simulink model "modelo_f_nico_local"  (R2024b)
settings: Solver=ode15s  StartTime=0.0  StopTime=600  FixedStep=0.001  RelTol=1e-3
InitFcn:
  | clc
  | clear
  | close all
  | parametros
  | gain_CL
  | calculo_observador_carro
  | calculo_observador_izaje
values from neighbouring files (symbols this model uses):
  b_cx = 1e6    (= 1000000)    [parametros.m]
  b_cy = 1e7    (= 10000000)    [parametros.m]
  b_ha = -(J_hEq + (r_hd/(2*i_h))*m_l) * w_des_h*(1 + n_h + n_h^2) + b_hEq    [gain_CL.m]
  b_hb = 1e8    (= 100000000)    [parametros.m]
  b_hd = 8    [parametros.m]
  b_hm = 18    [parametros.m]
  b_t = 90    [parametros.m]
  b_ta = M_tEq*w_des_t*(1+n_t+n_t^2)-b_tEq    [gain_CL.m]
  b_tb = 5e6    (= 5000000)    [parametros.m]
  b_td = 1.8    [parametros.m]
  b_tm = 6    [parametros.m]
  b_tw = 3e3    (= 3000)    [parametros.m]
  b_wu = 150    [parametros.m]
  g = 9.80665    [parametros.m]
  H_c = 2.59    [parametros.m]
  i_h = 22    [parametros.m]
  i_t = 30    [parametros.m]
  J_hd_hEb = 3800    [parametros.m]
  J_hm_hb = 30    [parametros.m]
  J_td = 1200    [parametros.m]
  J_tm_tb = 7    [parametros.m]
  K_cy = 1.8e9    (= 1800000000)    [parametros.m]
  k_hsa = -(J_hEq + (r_hd/(2*i_h))*m_l) * w_des_h^2*(n_h + n_h^2 + n_h^3)    [gain_CL.m]
  k_hsia = -(J_hEq + (r_hd/(2*i_h))*m_l) * n_h^3 * w_des_h^3    [gain_CL.m]
  k_tsa = M_tEq*w_des_t^2*n_t*(1+n_t+n_t^2)    [gain_CL.m]
  k_tsia = M_tEq*w_des_t^3*n_t^3    [gain_CL.m]
  K_tw = 4.8e5    (= 480000)    [parametros.m]
  k_wu = 2.36e8    (= 236000000)    [parametros.m]
  l_h_max = Y_t0-y_h_min    (= 65)    [parametros.m]
  l_h_maxE = l_h_max+0.5    (= 65.5)    [parametros.m]
  l_h_min = Y_t0-y_h_max    (= 5)    [parametros.m]
  l_h_minE = l_h_min-0.5    (= 4.5)    [parametros.m]
  Lt = place(At', Ct', polos_deseados)'    [calculo_observador_carro.m]
  M_cmax = 50000    [parametros.m]
  M_cmin = 2000    [parametros.m]
  M_s = 15000    [parametros.m]
  M_t = 30000    [parametros.m]
  r_hd = 0.75    [parametros.m]
  r_td = 0.50    (= 0.5)    [parametros.m]
  T_hbMax = 5e4    (= 50000)    [parametros.m]
  T_hEbMax = 1.1e6    (= 1100000)    [parametros.m]
  T_hmMax = 2e4    (= 20000)    [parametros.m]
  T_s = 0.001    [parametros.m]
  T_tbMax = 5e3    (= 5000)    [parametros.m]
  T_tmMax = 4e3    (= 4000)    [parametros.m]
  tau_tm = 1e-3    (= 0.001)    [parametros.m]
  tau_wl = 1 / (2 * pi * 2)    (= 0.0795774715459)    [parametros.m]
  theta_hm0 = -l_h0*i_h*2/r_hd    (= -2229.33333333)    [parametros.m]
  theta_tm0 = (x_t0)*i_t/r_td    (= -900)    [parametros.m]
  v_h_max_noload = 3    [parametros.m]
  v_lx0 = 0    [parametros.m]
  v_ly0 = 0    [parametros.m]
  v_t0 = 0    [parametros.m]
  v_t_max = 4    [parametros.m]
  W_c = ctrb(A, B_c(:,1))    [CyO_carro.m]    (also in CyO_izaje.m; parametros.m = 2.44)
  w_hm0 = 0    [parametros.m]
  w_hm_min_BRK = 999999999    [parametros.m]
  w_hm_rated = v_h_max_load*2*i_h/r_hd    (= 88)    [parametros.m]
  w_tm0 = (v_t0)*i_t/r_td    (= 0)    [parametros.m]
  w_tm_min_BRK = 999999999    [parametros.m]
  x_l0 = x_t0    (= -15)    [parametros.m]
  x_lidar_offset = 3.0    (= 3)    [parametros.m]
  x_t0 = -15    [parametros.m]
  x_t_max = 50    [parametros.m]
  x_t_maxE = x_t_max+0.5    (= 50.5)    [parametros.m]
  x_t_min = -30    [parametros.m]
  x_t_minE = x_t_min-0.5    (= -30.5)    [parametros.m]
  y_h_min = -20    [parametros.m]
  y_l0 = 7    [parametros.m]
  Y_sb = 5.0    (= 5)    [parametros.m]
  Y_t0 = 45    [parametros.m]
undefined symbols (not defined in the file or in its folder): carro_FC_safety_margin, izaje_FC_safety_margin, Lh
libraries: dspsigops x1, simulink x1
(part 1 of 2)
settings Model: Creator=nsorr  LastModifiedBy=nsorr
settings SolverCC: DecoupledContinuousIntegration=on

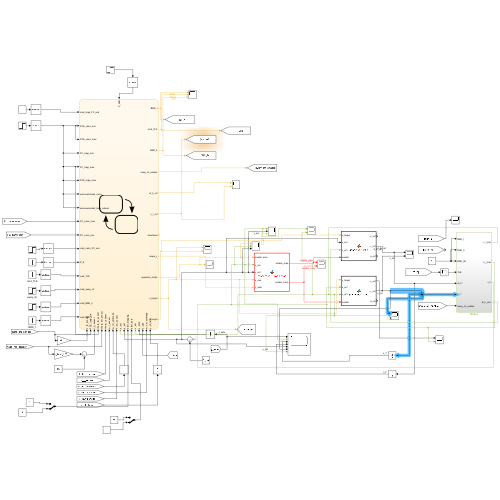
[thumbnail: Simulink's stored preview of the top-level diagram]
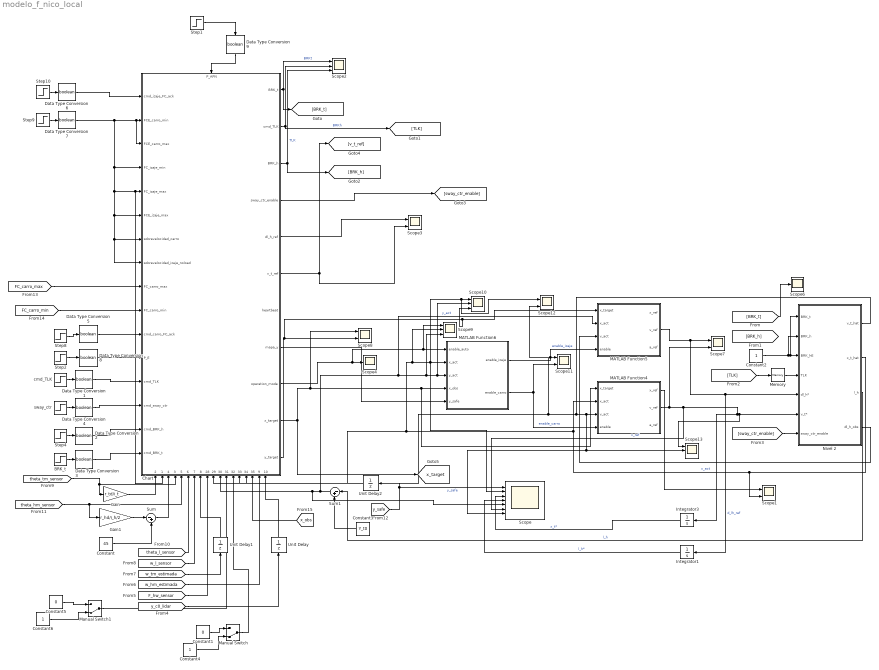
== system modelo_f_nico_local ==
  BRK_t : Step  Time=0  After=0  SampleTime=0
  Chart : Stateflow chart  TreatAsAtomicUnit=on
      settings: PortSchema="{\"entries\":[{\"content\":{\"sides\":[{\"content\":{\"connectorIds\":[\"In15\",\"In16\",\"In17\",\"In18\",\"In19\",\"In20\",\"In21\",\"In22\",\"In23\",\"In24\",\"In13\",\"In12\",\"In25\",\"In14\",\"In26\",\"In27\"]},\"type\":\"ConnectorPlacement.EquallySpacedRectSide\",\"uuid\":\"7880b9cd-08fb-4733-bb6b-48e405180dc5\"},{\"content\":{\"connectorIds\":[\"Out1\",\"Out3\",\"Out4\",\"Out5\",\"Out6\",\"Out2\",\"Out7\",\"Out8\",\"Out9\",\"Out10\",\"Out11\"],\"side\":\"RIGHT\"},\"type\":\"ConnectorPlacement.EquallySpacedRectSide\",\"uuid\":\"1a0088c7-0ec1-46fb-bd67-3069194311ce\"},{\"content\":{\"connectorIds\":[\"In11\"],\"side\":\"TOP\"},\"type\":\"ConnectorPlacement.EquallySpacedRectSide\",\"uuid\":\"63c24ea1-9c7d-47d6-85d5-bbef0a7be167\"},{\"content\":{\"connectorIds\":[\"In2\",\"In1\",\"In4\",\"In3\",\"In5\",\"In6\",\"In7\",\"In8\",\"In28\",\"In29\",\"In30\",\"In31\",\"In32\",\"In33\",\"In34\",\"In35\",\"In9\",\"In10\"],\"side\":\"BOTTOM\"},\"type\":\"ConnectorPlacement.EquallySpacedRectSide\",\"uuid\":\"56586e70-7155-4caa-800e-4bb67e399bfa\"}]},\"type\":\"ConnectorPlacement.EquallySpacedConnector\",\"uuid\":\"e7da0abc-eae0-41d9-ad4b-a3df1daa3702\"}],\"packageUris\":[\"http://schema.mathworks.com/mf0/Connector/R2020b\"],\"version\":\"1.0\"}"
  Constant : Constant  Value=45
  Constant1 : Constant  Value=0  OutDataTypeStr=boolean
  Constant2 : Constant
  Constant3 : Constant  Value=Y_t0
  Constant4 : Constant  OutDataTypeStr=boolean
  Constant5 : Constant  Value=0  OutDataTypeStr=boolean
  Constant6 : Constant  OutDataTypeStr=boolean
  Data Type Conversion{1..9} (9 alike) : DataTypeConversion  OutDataTypeStr=boolean  SaturateOnIntegerOverflow=off  RndMeth=Floor
  Gain : Gain  Gain=r_td/i_t
  Gain1 : Gain  Gain=r_hd/i_h/2
  Integrator1 : Integrator  InitialCondition=x_t0
  Integrator3 : Integrator  InitialCondition=x_t0
  MATLAB Function4 : MATLAB Function  TreatAsAtomicUnit=on  SystemSampleTime=T_s
  MATLAB Function5 : MATLAB Function  TreatAsAtomicUnit=on  SystemSampleTime=T_s
  MATLAB Function6 : MATLAB Function  TreatAsAtomicUnit=on  SystemSampleTime=T_s
  Manual Switch : ManualSwitch  CurrentSetting=0
  Manual Switch1 : ManualSwitch  CurrentSetting=0
  Memory : Memory
  Nivel 2 : Subsystem
  Scope : Scope  NumInputPorts=7
  Scope{1,3,7..8,11..12} (6 alike) : Scope  NumInputPorts=2
  Scope{2,9..10,13} (4 alike) : Scope  NumInputPorts=3
  Scope4 : Scope
  Scope6 : Scope
  Step1 : Step  SampleTime=0
  Step{4,8..10} (4 alike) : Step  Time=0  After=0  SampleTime=0
  Step2 : Step  Time=0  SampleTime=0
  Sum : Sum  Inputs=|-+
  Sum1 : Sum  Inputs=|-+
  Unit Delay : UnitDelay  SampleTime=T_s  HasFrameUpgradeWarning=on
  Unit Delay1 : UnitDelay  SampleTime=T_s  HasFrameUpgradeWarning=on
  Unit Delay2 : UnitDelay  SampleTime=T_s  HasFrameUpgradeWarning=on
  cmd_TLK : Step  Time=0  After=0  SampleTime=0
  sway_ctr : Step  Time=0  After=0  SampleTime=0
  tag scope: x_target=global
  wires:
  MATLAB Function5/2(v_ref) -> Scope7/1, Nivel 2/5(dl_h*), Integrator1/1  "d_lh_ref"
  Chart/9(operation_mode) -> Scope9/1, MATLAB Function6/1(enable_auto), Scope4/1
  Chart/1(BRK_t) -> [BRK_t], Scope2/1  "BRKt"
  [F_hw_sensor] -> Chart/28(F_hw_sensor)
  [theta_tm_sensor] -> Gain/1, Chart/3(theta_tm_sensor)
  [FC_carro_max] -> Chart/23(FC_carro_max)
  cmd_TLK/1 -> Data Type Conversion1/1
  Gain1/1 -> Sum/1
  Chart/6(dl_h_ref) -> Scope3/1
  Data Type Conversion7/1 -> Chart/17(FCE_carro_max), Chart/16(FCE_carro_min), Chart/18(FC_izaje_min), Chart/19(FC_izaje_max), Chart/1(FCE_izaje_min), Chart/22(sobrevelocidad_izaje_noload), Chart/21(sobrevelocidad_carro), Chart/20(FCE_izaje_max)
  Step2/1 -> Data Type Conversion8/1
  [theta_l_sensor] -> Chart/6(theta_l_sensor)
  Constant3/1 -> Sum1/2
  Chart/4(BRK_h) -> Scope2/3, [BRK_h]  "TLK"
  Data Type Conversion9/1 -> Chart/11(P_APN)
  Constant/1 -> Sum/2
  Gain/1 -> Chart/2(x_td_sensor)
  MATLAB Function6/2(enable_carro) -> Scope11/2, MATLAB Function4/4(enable)  "enable_carro"
  Data Type Conversion2/1 -> Chart/26(cmd_BRK_h)
  Step4/1 -> Data Type Conversion2/1
  [w_tm_estimada] -> Unit Delay1/1
  Manual Switch1/1 -> Chart/31(start_mapping)
  sway_ctr/1 -> Data Type Conversion4/1
  [w_hm_estimada] -> Chart/9(w_hm_estimada)
  Unit Delay1/1 -> Chart/8(w_tm_estimada)
  Sum1/1 -> MATLAB Function5/2(x_act), Scope10/2, MATLAB Function6/3(y_act), Scope9/3, Scope/5, Chart/30(y_act)  "y_act"
  Nivel 2/1(v_t_hat) -> Scope12/2, Chart/33(v_act), Scope13/2, Scope/7, MATLAB Function4/3(v_act)
  Chart/5(sway_ctr_enable) -> [sway_ctr_enable]
  [TLK] -> Memory/1
  [w_l_sensor] -> Chart/7(w_l_sensor)
  [BRK_t] -> Scope6/1
  Chart/2(v_t_ref) -> [v_t_ref], Scope3/2
  Data Type Conversion8/1 -> Chart/12(P_E)
  [theta_hm_sensor] -> Chart/5(theta_hm_sensor), Gain1/1
  Nivel 2/4(dl_h_obs) -> MATLAB Function5/3(v_act)
  Sum/1 -> Chart/4(l_h_sensor)
  [sway_ctr_enable] -> Nivel 2/7(sway_ctr_enable)
  Data Type Conversion1/1 -> Chart/25("cmd_TLK ")
  Nivel 2/3(l_h) -> Sum1/1  "l_h"
  Unit Delay/1 -> Chart/10(y_c0_lidar)
  Data Type Conversion5/1 -> Chart/13(cmd_carro_FC_ack)
  Nivel 2/2(x_t_hat) -> Scope1/2, MATLAB Function4/2(x_act), Chart/29(x_act), Scope12/1, Scope10/1, Scope/2, MATLAB Function6/2(x_act), Scope9/2  "x_act"
  Data Type Conversion6/1 -> Chart/15(cmd_izaje_FC_ack)
  Constant2/1 -> Nivel 2/1(BRK_t), Nivel 2/3(BRK_hE), Nivel 2/2(BRK_h)
  Step10/1 -> Data Type Conversion6/1
  MATLAB Function6/1(enable_izaje) -> MATLAB Function5/4(enable), Scope11/1  "enable_izaje"
  [y_c0_lidar] -> Unit Delay/1
  Chart/8(mapa_y) -> MATLAB Function6/5(y_safe)
  BRK_t/1 -> Data Type Conversion3/1
  Step8/1 -> Data Type Conversion5/1
  Chart/11(y_target) -> Scope8/2, Scope10/3, MATLAB Function5/1(x_target)
  Data Type Conversion4/1 -> Chart/14(cmd_sway_ctr)
  Step1/1 -> Data Type Conversion9/1
  Chart/10(x_target) -> Scope8/1, MATLAB Function4/1(x_target), MATLAB Function6/4(x_obs), [x_target]
  Data Type Conversion3/1 -> Chart/27(cmd_BRK_t)
  Step9/1 -> Data Type Conversion7/1
  Chart/3(cmd_TLK) -> [TLK], Scope2/2  "BRKh"
  MATLAB Function4/2(v_ref) -> Scope/6, Nivel 2/6(v_t*), Scope13/1, Integrator3/1, Scope7/2  "v_ref"
  [FC_carro_min] -> Chart/24(FC_carro_min)
  [y_safe] -> Unit Delay2/1, Scope/1  "y_safe"
  Unit Delay2/1 -> Chart/34(y_safe)
  Constant1/1 -> Manual Switch/1
  Constant4/1 -> Manual Switch/2
  Manual Switch/1 -> Chart/32(start_auto)
  Constant6/1 -> Manual Switch1/2
  Constant5/1 -> Manual Switch1/1
  Integrator3/1 -> Scope/3  "x_t*"
  Integrator1/1 -> Scope/4  "l_h*"
  [x_obs] -> Chart/35(x_obs)
  Memory/1 -> Nivel 2/4(TLK)
  MATLAB Function4/1(x_ref) -> Scope1/1

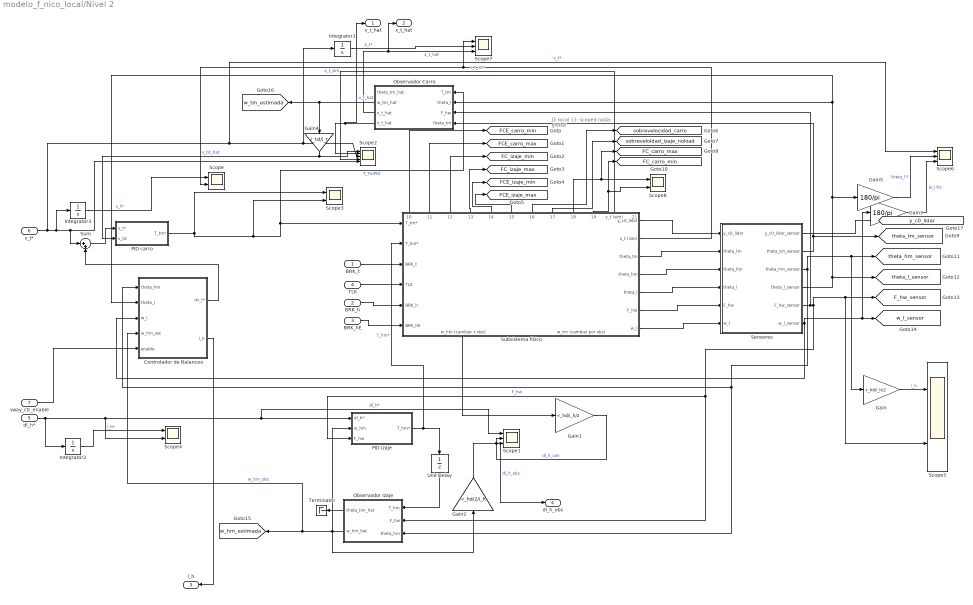
== system modelo_f_nico_local/Nivel 2 ==
  note: []: local
      | {}: scoped
      | nada: global
  BRK_t : Inport
  BRK_h : Inport  Port=2
  BRK_hE : Inport  Port=3
  TLK : Inport  Port=4
  dl_h* : Inport  Port=5
  v_t* : Inport  Port=6
  sway_ctr_enable : Inport  Port=7
  Controlador de Balanceo : Subsystem
  Gain : Gain  Gain=-r_hd/i_h/2
  Gain1 : Gain  Gain=-r_hd/i_h/2
  Gain2 : Gain  Gain=-r_hd/2/i_h
  Gain3 : Gain  Gain=180/pi
  Gain4 : Gain  Gain=r_td/i_t
  Gain5 : Gain  Gain=180/pi
  Integrator1 : Integrator  InitialCondition=x_t0
  Integrator2 : Integrator
  Integrator3 : Integrator  InitialCondition=x_t0
  Observador Carro : Subsystem
  Observador Izaje : Subsystem
  PID carro : Subsystem
  PID izaje : Subsystem
  Scope{,3..5,8} (5 alike) : Scope  NumInputPorts=2
  Scope1 : Scope  NumInputPorts=3
  Scope2 : Scope  NumInputPorts=5
  Scope6 : Scope  NumInputPorts=3
  Scope7 : Scope  NumInputPorts=3
  Sensores : Subsystem
  Subsistema físico : Subsystem
      settings: PortSchema="{\"entries\":[{\"content\":{\"sides\":[{\"content\":{\"connectorIds\":[\"In1\",\"In2\",\"In3\",\"In4\",\"In5\",\"In6\"]},\"type\":\"ConnectorPlacement.EquallySpacedRectSide\",\"uuid\":\"aa1cb789-2051-45a4-8cb8-6dd2078290cc\"},{\"content\":{\"connectorIds\":[\"Out1\",\"Out2\",\"Out3\",\"Out4\",\"Out5\",\"Out6\",\"Out7\"],\"side\":\"RIGHT\"},\"type\":\"ConnectorPlacement.EquallySpacedRectSide\",\"uuid\":\"7fe62279-dd3b-46db-ba9e-e4633dcea5c6\"},{\"content\":{\"connectorIds\":[\"Out10\",\"Out11\",\"Out12\",\"Out13\",\"Out14\",\"Out15\",\"Out16\",\"Out17\",\"Out18\",\"Out19\",\"Out20\",\"Out21\"],\"side\":\"TOP\"},\"type\":\"ConnectorPlacement.EquallySpacedRectSide\",\"uuid\":\"a5663ea7-10d8-47d7-b8ed-8fbfb239b85a\"},{\"content\":{\"connectorIds\":[\"Out8\",\"Out9\"],\"side\":\"BOTTOM\"},\"type\":\"ConnectorPlacement.EquallySpacedRectSide\",\"uuid\":\"9ec9131f-7b2f-42d7-8a86-9462c3c282b3\"}]},\"type\":\"ConnectorPlacement.EquallySpacedConnector\",\"uuid\":\"e7df1a56-7803-4e0d-8bf9-081877eb8c08\"}],\"packageUris\":[\"http://schema.mathworks.com/mf0/Connector/R2020b\"],\"version\":\"1.0\"}"
  Sum : Sum  Inputs=|++
  Terminator : Terminator
  Unit Delay : UnitDelay  SampleTime=T_s  HasFrameUpgradeWarning=on
  v_t_hat : Outport
  x_t_hat : Outport  Port=2
  l_h : Outport  Port=3
  dl_h_obs : Outport  Port=4
  tag scope: FCE_carro_max=global, FCE_carro_min=global, FCE_izaje_max=global, FCE_izaje_min=global, FC_carro_max=global, FC_carro_min=global, FC_izaje_max=global, FC_izaje_min=global, F_hw_sensor=global, sobrevelocidad_carro=global, sobreveloidad_izaje_noload=global, theta_hm_sensor=global, theta_l_sensor=global, theta_tm_sensor=global, w_hm_estimada=global, w_l_sensor=global, w_tm_estimada=global, y_c0_lidar=global
  wires:
  Subsistema físico/2(x_t (sim)) -> Scope7/1, Scope/2  "x_t_sim"
  Sensores/5(F_hw_sensor) -> Observador Izaje/2(F_hw), PID izaje/3(F_hw), Scope5/2, [F_hw_sensor], Observador Carro/3(F_hw)  "F_hw"
  v_t*/1 -> Scope2/5, Sum/1, Integrator3/1, Scope6/1, Integrator1/1, Scope2/3  "v_t*"
  Sensores/2(theta_tm_sensor) -> Observador Carro/4(theta_tm), [theta_tm_sensor]
  Subsistema físico/18(FC_carro_max) -> Scope8/1, [FC_carro_max]
  Sensores/3(theta_hm_sensor) -> Gain/1, [theta_hm_sensor], Observador Izaje/3(theta_hm), Controlador de Balanceo/1(theta_hm)
  Integrator3/1 -> Scope/1  "x_t*"
  Gain/1 -> Scope5/1  "l_h"
  Sensores/6(w_l_sensor) -> Gain3/1, [w_l_sensor], Controlador de Balanceo/3(w_l)
  PID carro/1(T_tm*) -> Scope3/2, Observador Carro/1(T_tm), Subsistema físico/1(T_tm*), Scope3/1  "T_TmPID"
  Subsistema físico/14(FCE_izaje_min) -> [FCE_izaje_min]
  Unit Delay/1 -> Observador Izaje/1(T_hm)
  Subsistema físico/12(FC_izaje_min) -> [FC_izaje_min]
  Subsistema físico/15(FCE_izaje_max) -> [FCE_izaje_max]
  Observador Izaje/2(w_hm_hat) -> Gain2/1, Controlador de Balanceo/4(w_hm_est), [w_hm_estimada], PID izaje/2(w_hm)  "w_hm_obs"
  PID izaje/1(T_hm*) -> Unit Delay/1, Subsistema físico/2(T_hm*)  "T_hm*"
  Subsistema físico/7(w_l) -> Sensores/6(w_l)
  Subsistema físico/16(sobrevelocidad_carro) -> [sobrevelocidad_carro]
  Subsistema físico/4(theta_hm) -> Sensores/3(theta_hm)
  Gain1/1 -> Scope1/2  "dl_h_sim"
  Observador Izaje/1(theta_hm_hat) -> Terminator/1
  dl_h*/1 -> Integrator2/1, Scope4/2, Scope1/1, PID izaje/1(dl_h*)  "dl_h*"
  Gain2/1 -> dl_h_obs/1, Scope1/3  "dl_h_obs"
  Subsistema físico/1(y_c0_lidar) -> Sensores/1(y_c0_lidar)
  Subsistema físico/6(F_hw) -> Sensores/5(F_hw)
  Subsistema físico/3(theta_tm) -> Sensores/2(theta_tm)
  Subsistema físico/17(sobrevelocidad_izaje_noload) -> [sobreveloidad_izaje_noload]
  Subsistema físico/8(w_hm (cambiar x obs)) -> Gain1/1
  Integrator2/1 -> Scope4/1  "l_h*"
  Integrator1/1 -> Scope7/2  "x_t*"
  Subsistema físico/10(FCE_carro_min) -> [FCE_carro_min]
  Sensores/4(theta_l_sensor) -> Observador Carro/2(theta_l), Controlador de Balanceo/2(theta_l), Gain5/1, [theta_l_sensor]
  Subsistema físico/5(theta_l) -> Sensores/4(theta_l)
  Subsistema físico/13(FC_izaje_max) -> [FC_izaje_max]
  Subsistema físico/19(FC_carro_min) -> Scope8/2, [FC_carro_min]
  Subsistema físico/11(FCE_carro_max) -> [FCE_carro_max]
  Gain5/1 -> Scope6/2  "theta_l º"
  BRK_t/1 -> Subsistema físico/3(BRK_t)
  BRK_h/1 -> Subsistema físico/5(BRK_h)
  BRK_hE/1 -> Subsistema físico/6(BRK_hE)
  TLK/1 -> Subsistema físico/4(TLK)
  Sensores/1(y_c0_lidar_sensor) -> [y_c0_lidar]
  sway_ctr_enable/1 -> Controlador de Balanceo/5(enable)
  Observador Carro/2(w_tm_hat) -> [w_tm_estimada], Gain4/1
  Subsistema físico/20(v_t (sim)) -> Scope2/4  "v_t_sim"
  Gain4/1 -> PID carro/2(v_td), Scope2/1  "v_td_hat"
  Observador Carro/3(x_t_hat) -> Scope7/3, x_t_hat/1  "x_t_hat"
  Observador Carro/4(v_t_hat) -> v_t_hat/1, Scope2/2  "v_t_hat"
  Controlador de Balanceo/1(dv_t*) -> Sum/2
  Gain3/1 -> Scope6/3  "w_l º/s"
  Controlador de Balanceo/2(l_h) -> l_h/1
  Sum/1 -> PID carro/1(v_t*)

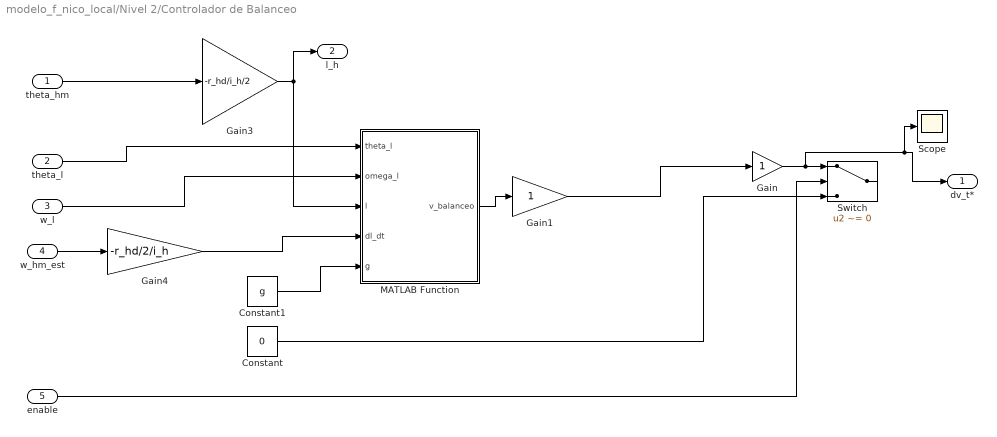
== system modelo_f_nico_local/Nivel 2/Controlador de Balanceo ==
  theta_hm : Inport
  theta_l : Inport  Port=2
  w_l : Inport  Port=3
  w_hm_est : Inport  Port=4
  enable : Inport  Port=5
  Constant : Constant  Value=0
  Constant1 : Constant  Value=g
  Gain : Gain
  Gain1 : Gain
  Gain3 : Gain  Gain=-r_hd/i_h/2
  Gain4 : Gain  Gain=-r_hd/2/i_h
  MATLAB Function : MATLAB Function  TreatAsAtomicUnit=on  SystemSampleTime=T_s
  Scope : Scope
  Switch : Switch  Criteria=u2 ~= 0  SaturateOnIntegerOverflow=off  InputSameDT=off
  dv_t* : Outport
  l_h : Outport  Port=2
  wires:
  w_hm_est/1 -> Gain4/1
  theta_hm/1 -> Gain3/1
  Gain1/1 -> Gain/1
  Constant/1 -> Switch/3
  Gain/1 -> Scope/1, dv_t*/1, Switch/1
  MATLAB Function/1(v_balanceo) -> Gain1/1
  enable/1 -> Switch/2
  theta_l/1 -> MATLAB Function/1(theta_l)
  w_l/1 -> MATLAB Function/2(omega_l)
  Gain3/1 -> l_h/1, MATLAB Function/3(l)
  Constant1/1 -> MATLAB Function/5(g)
  Gain4/1 -> MATLAB Function/4(dl_dt)

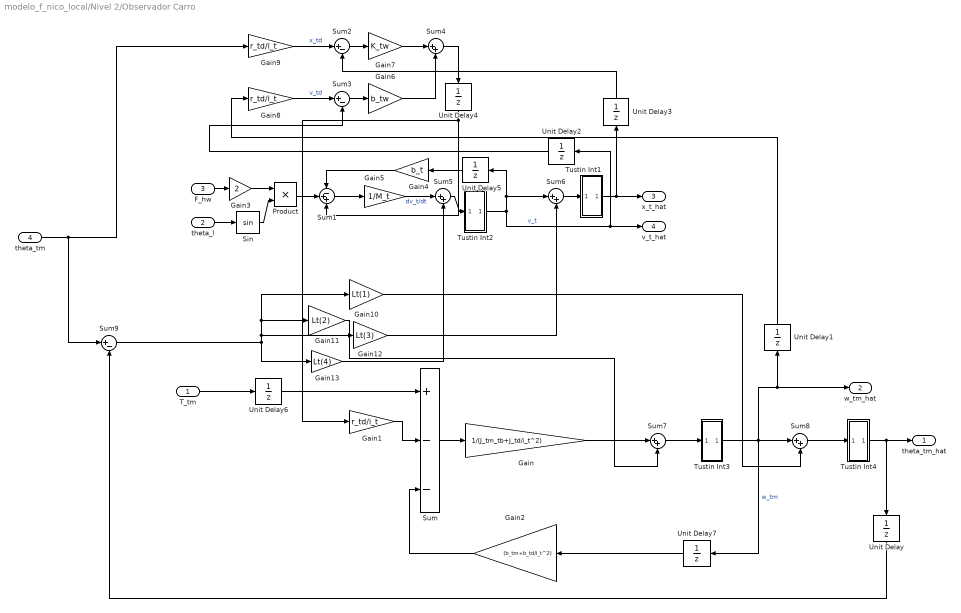
== system modelo_f_nico_local/Nivel 2/Observador Carro ==
  T_tm : Inport
  theta_l : Inport  Port=2
  F_hw : Inport  Port=3
  theta_tm : Inport  Port=4
  Gain : Gain  Gain=1/(J_tm_tb+J_td/i_t^2)
  Gain1 : Gain  Gain=r_td/i_t
  Gain10 : Gain  Gain=Lt(1)
  Gain11 : Gain  Gain=Lt(2)
  Gain12 : Gain  Gain=Lt(3)
  Gain13 : Gain  Gain=Lt(4)
  Gain2 : Gain  Gain=(b_tm+b_td/i_t^2)
  Gain3 : Gain  Gain=2
  Gain4 : Gain  Gain=b_t
  Gain5 : Gain  Gain=1/M_t
  Gain6 : Gain  Gain=b_tw
  Gain7 : Gain  Gain=K_tw
  Gain8 : Gain  Gain=r_td/i_t
  Gain9 : Gain  Gain=r_td/i_t
  Product : Product
  Sin : Trigonometry
  Sum : Sum  Inputs=+--
  Sum1 : Sum  Inputs=-++
  Sum2 : Sum  Inputs=|+-
  Sum3 : Sum  Inputs=|+-
  Sum{4..8} (5 alike) : Sum  Inputs=|++
  Sum9 : Sum  Inputs=|+-
  Tustin Int1 : Subsystem
  Tustin Int2 : Subsystem
  Tustin Int3 : Subsystem
  Tustin Int4 : Subsystem
  Unit Delay : UnitDelay  InitialCondition=theta_tm0  SampleTime=T_s  HasFrameUpgradeWarning=on
  Unit Delay{1..2,4..6} (5 alike) : UnitDelay  SampleTime=T_s  HasFrameUpgradeWarning=on
  Unit Delay3 : UnitDelay  InitialCondition=theta_tm0*r_td/i_t  SampleTime=T_s  HasFrameUpgradeWarning=on
  Unit Delay7 : UnitDelay  InitialCondition=theta_tm0  SampleTime=T_s  HasFrameUpgradeWarning=on
  theta_tm_hat : Outport
  w_tm_hat : Outport  Port=2
  x_t_hat : Outport  Port=3
  v_t_hat : Outport  Port=4
  wires:
  Sum/1 -> Gain/1
  Gain1/1 -> Sum/2
  Sum4/1 -> Unit Delay4/1
  Gain2/1 -> Sum/3
  Tustin Int3/1(Out1) -> Sum8/1, Unit Delay1/1, w_tm_hat/1, Unit Delay7/1  "w_tm"
  Gain/1 -> Sum7/1
  Tustin Int4/1(Out1) -> Unit Delay/1, theta_tm_hat/1
  theta_l/1 -> Sin/1
  Sin/1 -> Product/2
  Product/1 -> Sum1/2
  Gain3/1 -> Product/1
  Sum1/1 -> Gain5/1
  Tustin Int2/1(Out1) -> Unit Delay5/1, Sum6/1, v_t_hat/1, Unit Delay2/1  "v_t"
  Gain4/1 -> Sum1/1
  Tustin Int1/1(Out1) -> Unit Delay3/1, x_t_hat/1
  Gain5/1 -> Sum5/1  "dv_t/dt"
  F_hw/1 -> Gain3/1
  Gain7/1 -> Sum4/1
  Gain6/1 -> Sum4/2
  Sum3/1 -> Gain6/1
  Gain9/1 -> Sum2/1  "x_td"
  theta_tm/1 -> Sum9/1, Gain9/1
  Sum2/1 -> Gain7/1
  Gain8/1 -> Sum3/1  "v_td"
  Sum5/1 -> Tustin Int2/1(In1)
  Sum6/1 -> Tustin Int1/1(In1)
  Sum8/1 -> Tustin Int4/1(In1)
  Sum7/1 -> Tustin Int3/1(In1)
  Sum9/1 -> Gain12/1, Gain11/1, Gain10/1, Gain13/1
  Gain10/1 -> Sum8/2
  Gain11/1 -> Sum7/2
  Gain12/1 -> Sum6/2
  Gain13/1 -> Sum5/2
  Unit Delay/1 -> Sum9/2
  Unit Delay1/1 -> Gain8/1
  Unit Delay2/1 -> Sum3/2
  Unit Delay3/1 -> Sum2/2
  Unit Delay4/1 -> Gain1/1, Sum1/3
  T_tm/1 -> Unit Delay6/1
  Unit Delay5/1 -> Gain4/1
  Unit Delay6/1 -> Sum/1
  Unit Delay7/1 -> Gain2/1

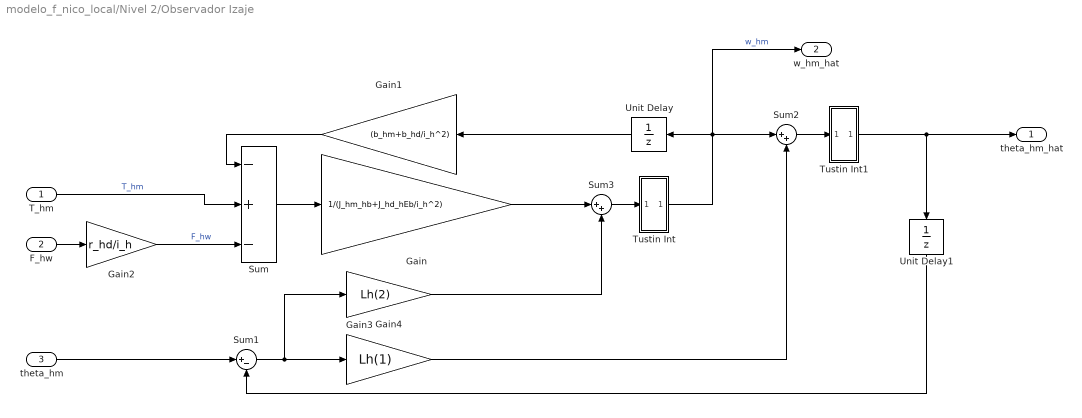
== system modelo_f_nico_local/Nivel 2/Observador Izaje ==
  T_hm : Inport
  F_hw : Inport  Port=2
  theta_hm : Inport  Port=3
  Gain : Gain  Gain=1/(J_hm_hb+J_hd_hEb/i_h^2)
  Gain1 : Gain  Gain=(b_hm+b_hd/i_h^2)
  Gain2 : Gain  Gain=r_hd/i_h
  Gain3 : Gain  Gain=Lh(1)
  Gain4 : Gain  Gain=Lh(2)
  Sum : Sum  Inputs=-+-
  Sum1 : Sum  Inputs=|+-
  Sum2 : Sum  Inputs=|++
  Sum3 : Sum  Inputs=|++
  Tustin Int : Subsystem
  Tustin Int1 : Subsystem
  Unit Delay : UnitDelay  SampleTime=T_s  HasFrameUpgradeWarning=on
  Unit Delay1 : UnitDelay  InitialCondition=theta_hm0  SampleTime=T_s  HasFrameUpgradeWarning=on
  theta_hm_hat : Outport
  w_hm_hat : Outport  Port=2
  wires:
  F_hw/1 -> Gain2/1
  Gain1/1 -> Sum/1
  Gain/1 -> Sum3/1
  Sum/1 -> Gain/1
  T_hm/1 -> Sum/2  "T_hm"
  Tustin Int/1(Out1) -> Sum2/1, w_hm_hat/1, Unit Delay/1  "w_hm"
  Tustin Int1/1(Out1) -> Unit Delay1/1, theta_hm_hat/1
  Gain2/1 -> Sum/3  "F_hw"
  theta_hm/1 -> Sum1/1
  Sum1/1 -> Gain4/1, Gain3/1
  Gain3/1 -> Sum2/2
  Sum2/1 -> Tustin Int1/1(In1)
  Sum3/1 -> Tustin Int/1(In1)
  Gain4/1 -> Sum3/2
  Unit Delay/1 -> Gain1/1
  Unit Delay1/1 -> Sum1/2

== system modelo_f_nico_local/Nivel 2/PID carro ==
  note: Este PID no está diseñado para manejar la resonancia que incluye el lazo de v_t por lo que alimentarlo con v_t excitaría dicho modo e inestabilizaría la planta.
  v_t* : Inport
  v_td : Inport  Port=2
  Gain : Gain  Gain=b_ta
  Gain1 : Gain  Gain=k_tsia
  Gain2 : Gain  Gain=k_tsa
  Sum : Sum  Inputs=|+-
  Sum1 : Sum  Inputs=+++
  Tustin Int1 : Subsystem
  Tustin Int2 : Subsystem
  T_tm* : Outport
  wires:
  Gain2/1 -> Sum1/2  "P"
  v_t*/1 -> Sum/1
  Sum1/1 -> T_tm*/1
  Sum/1 -> Gain/1, Tustin Int2/1(In1)  "e"
  Tustin Int2/1(Out1) -> Tustin Int1/1(In1), Gain2/1
  Tustin Int1/1(Out1) -> Gain1/1
  v_td/1 -> Sum/2
  Gain/1 -> Sum1/3  "D"
  Gain1/1 -> Sum1/1  "I"

== system modelo_f_nico_local/Nivel 2/PID izaje ==
  dl_h* : Inport
  w_hm : Inport  Port=2
  F_hw : Inport  Port=3
  Gain : Gain  Gain=b_ha
  Gain1 : Gain  Gain=k_hsia
  Gain2 : Gain  Gain=k_hsa
  Gain3 : Gain  Gain=-r_hd/2/i_h
  Gain4 : Gain  Gain=r_hd/(2*i_h)
  Sum : Sum  Inputs=|+-
  Sum1 : Sum  Inputs=+++
  Sum2 : Sum  Inputs=|++
  Tustin Int1 : Subsystem
  Tustin Int2 : Subsystem
  T_hm* : Outport
  wires:
  Gain2/1 -> Sum1/2  "P"
  dl_h*/1 -> Sum/1
  Gain/1 -> Sum1/3  "D"
  Gain1/1 -> Sum1/1  "I"
  w_hm/1 -> Gain3/1
  Sum1/1 -> Sum2/1
  Sum/1 -> Tustin Int1/1(In1), Gain/1
  Tustin Int1/1(Out1) -> Tustin Int2/1(In1), Gain2/1
  Tustin Int2/1(Out1) -> Gain1/1
  Gain3/1 -> Sum/2
  Sum2/1 -> T_hm*/1
  Gain4/1 -> Sum2/2
  F_hw/1 -> Gain4/1

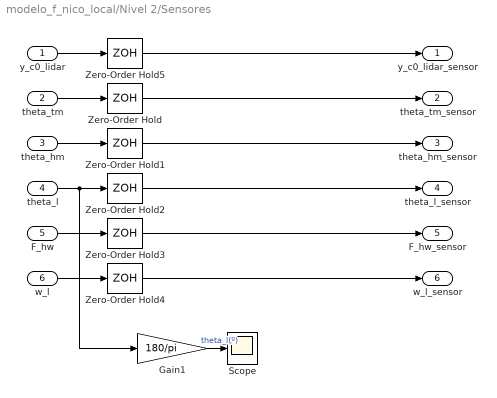
== system modelo_f_nico_local/Nivel 2/Sensores ==
  y_c0_lidar : Inport
  theta_tm : Inport  Port=2
  theta_hm : Inport  Port=3
  theta_l : Inport  Port=4
  F_hw : Inport  Port=5
  w_l : Inport  Port=6
  Gain1 : Gain  Gain=180/pi
  Scope : Scope
  Zero-Order Hold{,1..5} (6 alike) : ZeroOrderHold  SampleTime=T_s
  y_c0_lidar_sensor : Outport
  theta_tm_sensor : Outport  Port=2
  theta_hm_sensor : Outport  Port=3
  theta_l_sensor : Outport  Port=4
  F_hw_sensor : Outport  Port=5
  w_l_sensor : Outport  Port=6
  wires:
  theta_tm/1 -> Zero-Order Hold/1
  Zero-Order Hold/1 -> theta_tm_sensor/1
  Zero-Order Hold1/1 -> theta_hm_sensor/1
  theta_hm/1 -> Zero-Order Hold1/1
  w_l/1 -> Zero-Order Hold4/1
  F_hw/1 -> Zero-Order Hold3/1
  theta_l/1 -> Gain1/1, Zero-Order Hold2/1
  Zero-Order Hold2/1 -> theta_l_sensor/1
  Zero-Order Hold3/1 -> F_hw_sensor/1
  Zero-Order Hold4/1 -> w_l_sensor/1
  Gain1/1 -> Scope/1  "theta_l(º)"
  Zero-Order Hold5/1 -> y_c0_lidar_sensor/1
  y_c0_lidar/1 -> Zero-Order Hold5/1

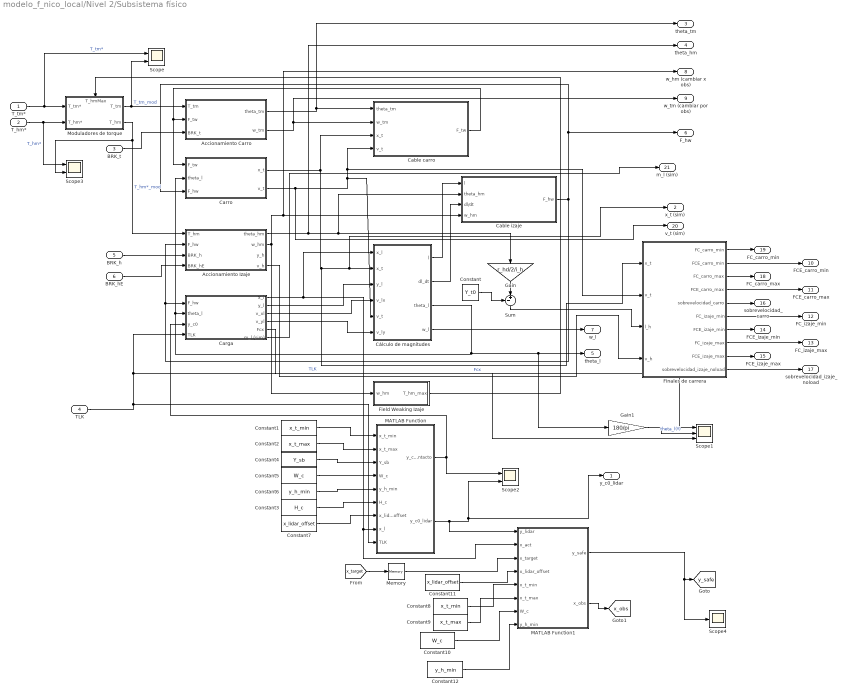
== system modelo_f_nico_local/Nivel 2/Subsistema físico ==
  T_tm* : Inport
  T_hm* : Inport  Port=2
  BRK_t : Inport  Port=3
  TLK : Inport  Port=4
  BRK_h : Inport  Port=5
  BRK_hE : Inport  Port=6
  Accionamiento Carro : Subsystem
  Accionamiento Izaje : Subsystem
  Cable carro : Subsystem
  Cable izaje : Subsystem
  Carga : Subsystem
  Carro : Subsystem
  Constant : Constant  Value=Y_t0
  Constant1 : Constant  Value=x_t_min
  Constant10 : Constant  Value=W_c
  Constant11 : Constant  Value=x_lidar_offset
  Constant12 : Constant  Value=y_h_min
  Constant2 : Constant  Value=x_t_max
  Constant3 : Constant  Value=H_c
  Constant4 : Constant  Value=Y_sb
  Constant5 : Constant  Value=W_c
  Constant6 : Constant  Value=y_h_min
  Constant7 : Constant  Value=x_lidar_offset
  Constant8 : Constant  Value=x_t_min
  Constant9 : Constant  Value=x_t_max
  Cálculo de magnitudes : Subsystem
  Field Weaking Izaje : Subsystem
  Finales de carrera : Subsystem
  Gain : Gain  Gain=r_hd/2/i_h
  Gain1 : Gain  Gain=180/pi
  MATLAB Function : MATLAB Function  TreatAsAtomicUnit=on  SystemSampleTime=T_s
  MATLAB Function1 : MATLAB Function  TreatAsAtomicUnit=on  SystemSampleTime=T_s
  Memory : Memory
  Moduladores de torque : Subsystem
      settings: PortSchema="{\"entries\":[{\"content\":{\"sides\":[{\"content\":{\"connectorIds\":[\"In1\",\"In2\"]},\"type\":\"ConnectorPlacement.EquallySpacedRectSide\",\"uuid\":\"c66d3892-523c-433a-8dde-517eb495bac1\"},{\"content\":{\"connectorIds\":[\"Out1\",\"Out2\"],\"side\":\"RIGHT\"},\"type\":\"ConnectorPlacement.EquallySpacedRectSide\",\"uuid\":\"bbb0a9b0-6ff9-4fa8-ace8-11da5b7abadd\"},{\"content\":{\"connectorIds\":[\"In3\"],\"side\":\"TOP\"},\"type\":\"ConnectorPlacement.EquallySpacedRectSide\",\"uuid\":\"35baaaad-8e6c-401a-84f7-749de5492b29\"}]},\"type\":\"ConnectorPlacement.EquallySpacedConnector\",\"uuid\":\"d8d05b6c-004b-40f1-854a-ea077232777a\"}],\"packageUris\":[\"http://schema.mathworks.com/mf0/Connector/R2020b\"],\"version\":\"1.0\"}"
  Scope : Scope  NumInputPorts=2
  Scope1 : Scope  NumInputPorts=3
  Scope2 : Scope  NumInputPorts=2
  Scope3 : Scope  NumInputPorts=2
  Scope4 : Scope
  Sum : Sum  Inputs=-+|
  y_c0_lidar : Outport
  x_t (sim) : Outport  Port=2
  theta_tm : Outport  Port=3
  theta_hm : Outport  Port=4
  theta_l : Outport  Port=5
  F_hw : Outport  Port=6
  w_l : Outport  Port=7
  w_hm (cambiar x obs) : Outport  Port=8
  w_tm (cambiar por obs) : Outport  Port=9
  FCE_carro_min : Outport  Port=10
  FCE_carro_max : Outport  Port=11
  FC_izaje_min : Outport  Port=12
  FC_izaje_max : Outport  Port=13
  FCE_izaje_min : Outport  Port=14
  FCE_izaje_max : Outport  Port=15
  sobrevelocidad_carro : Outport  Port=16
  sobrevelocidad_izaje_noload : Outport  Port=17
  FC_carro_max : Outport  Port=18
  FC_carro_min : Outport  Port=19
  v_t (sim) : Outport  Port=20
  m_l (sim) : Outport  Port=21
  tag scope: x_obs=global, y_safe=global
  wires:
  T_tm*/1 -> Scope/1, Moduladores de torque/1(T_tm*)  "T_tm*"
  Accionamiento Carro/1(theta_tm) -> theta_tm/1, Cable carro/1(theta_tm)
  Accionamiento Carro/2(w_tm) -> w_tm (cambiar por obs)/1, Cable carro/2(w_tm)
  Carro/1(x_t) -> Finales de carrera/1(x_t), x_t (sim)/1, Cálculo de magnitudes/2(x_t), Cable carro/3(x_t)
  Carro/2(v_t) -> v_t (sim)/1, Cálculo de magnitudes/5(v_t), Cable carro/4(v_t), Finales de carrera/2(v_t)
  Cable carro/1(F_tw) -> Carro/1(F_tw), Accionamiento Carro/2(F_tw)
  Carga/1(x_l) -> MATLAB Function1/2(x_act), MATLAB Function/8(x_l), Cálculo de magnitudes/1(x_l)
  Carga/2(y_l) -> Cálculo de magnitudes/3(y_l)
  Carga/3(v_xl) -> Cálculo de magnitudes/4(v_lx)
  Carga/4(v_yl) -> Cálculo de magnitudes/6(v_ly)
  Cálculo de magnitudes/1(l) -> Cable izaje/1(l)
  Accionamiento Izaje/1(theta_hm) -> Gain/1, Cable izaje/2(theta_hm), theta_hm/1
  Cable izaje/1(F_hw) -> F_hw/1, Carro/3(F_hw), Accionamiento Izaje/2(F_hw), Carga/1(F_hw)
  Cálculo de magnitudes/2(dl_dt) -> Cable izaje/3(dl/dt)
  T_hm*/1 -> Scope3/1, Moduladores de torque/2(T_hm*)  "T_hm*"
  Accionamiento Izaje/2(w_hm) -> w_hm (cambiar x obs)/1, Cable izaje/4(w_hm), Field Weaking Izaje/1(w_hm)
  BRK_t/1 -> Accionamiento Carro/3(BRK_t)
  BRK_h/1 -> Accionamiento Izaje/3(BRK_h)
  BRK_hE/1 -> Accionamiento Izaje/4(BRK_hE)
  TLK/1 -> Scope1/3, Carga/4(TLK), MATLAB Function/9(TLK)  "TLK"
  Accionamiento Izaje/4(v_h) -> Finales de carrera/4(v_h)
  Cálculo de magnitudes/4(w_l) -> w_l/1
  Moduladores de torque/1(T_tm) -> Scope/2, Accionamiento Carro/1(T_tm)  "T_tm_mod"
  Field Weaking Izaje/1(T_hm_max) -> Moduladores de torque/3(T_hmMax)
  Moduladores de torque/2(T_hm) -> Scope3/2, Accionamiento Izaje/1(T_hm)  "T_hm*_mod"
  Finales de carrera/1(FC_carro_min) -> FC_carro_min/1
  Finales de carrera/2(FCE_carro_min) -> FCE_carro_min/1
  Finales de carrera/3(FC_carro_max) -> FC_carro_max/1
  Finales de carrera/4(FCE_carro_max) -> FCE_carro_max/1
  Finales de carrera/5(sobrevelocidad_carro) -> sobrevelocidad_carro/1
  Finales de carrera/7(FCE_izaje_min) -> FCE_izaje_min/1
  Finales de carrera/6(FC_izaje_min) -> FC_izaje_min/1
  Finales de carrera/8(FC_izaje_max) -> FC_izaje_max/1
  Finales de carrera/9(FCE_izaje_max) -> FCE_izaje_max/1
  Finales de carrera/10(sobrevelocidad_izaje_noload) -> sobrevelocidad_izaje_noload/1
  Constant1/1 -> MATLAB Function/1(x_t_min)
  Constant2/1 -> MATLAB Function/2(x_t_max)
  Constant3/1 -> MATLAB Function/6(H_c)
  Constant4/1 -> MATLAB Function/3(Y_sb)
  Constant5/1 -> MATLAB Function/4(W_c)
  Constant6/1 -> MATLAB Function/5(y_h_min)
  MATLAB Function/1(y_c0_contacto) -> Carga/3(y_c0), Scope2/1
  Constant7/1 -> MATLAB Function/7(x_lidar_offset)
  MATLAB Function/2(y_c0_lidar) -> MATLAB Function1/1(y_lidar), Scope2/2, y_c0_lidar/1
  Carga/5(Fcx) -> Scope1/1  "Fcx"
  Gain1/1 -> Scope1/2  "theta_l(º)"
  Sum/1 -> Finales de carrera/3(l_h)
  Gain/1 -> Sum/2
  Constant/1 -> Sum/1
  Cálculo de magnitudes/3(theta_l) -> Carro/2(theta_l), Carga/2(theta_l), Gain1/1, theta_l/1
  Carga/6(m_l (sim)) -> m_l (sim)/1
  [x_target] -> Memory/1
  MATLAB Function1/1(y_safe) -> Scope4/1, [y_safe]
  Constant11/1 -> MATLAB Function1/4(x_lidar_offset)
  Constant8/1 -> MATLAB Function1/5(x_t_min)
  Constant9/1 -> MATLAB Function1/6(x_t_max)
  Constant10/1 -> MATLAB Function1/7(W_c)
  Constant12/1 -> MATLAB Function1/8(y_h_min)
  MATLAB Function1/2(x_obs) -> [x_obs]
  Memory/1 -> MATLAB Function1/3(x_target)

== system modelo_f_nico_local/Nivel 2/Observador Carro/Tustin Int1 ==
  In1 : Inport
  Gain : Gain  Gain=T_s/2
  Sum : Sum  Inputs=|++
  Sum1 : Sum  Inputs=|++
  Unit Delay : UnitDelay  InitialCondition=theta_tm0*r_td/i_t  SampleTime=T_s  HasFrameUpgradeWarning=on
  Unit Delay1 : UnitDelay  SampleTime=T_s  HasFrameUpgradeWarning=on
  Out1 : Outport
  wires:
  Sum1/1 -> Unit Delay/1, Out1/1
  Unit Delay/1 -> Sum1/2
  Unit Delay1/1 -> Sum/2
  In1/1 -> Sum/1, Unit Delay1/1
  Sum/1 -> Gain/1
  Gain/1 -> Sum1/1

== system modelo_f_nico_local/Nivel 2/Observador Carro/Tustin Int2 ==
  In1 : Inport
  Gain : Gain  Gain=T_s/2
  Sum : Sum  Inputs=|++
  Sum1 : Sum  Inputs=|++
  Unit Delay : UnitDelay  SampleTime=T_s  HasFrameUpgradeWarning=on
  Unit Delay1 : UnitDelay  SampleTime=T_s  HasFrameUpgradeWarning=on
  Out1 : Outport
  wires:
  Sum1/1 -> Unit Delay/1, Out1/1
  Unit Delay/1 -> Sum1/2
  Unit Delay1/1 -> Sum/2
  In1/1 -> Sum/1, Unit Delay1/1
  Sum/1 -> Gain/1
  Gain/1 -> Sum1/1

== system modelo_f_nico_local/Nivel 2/Observador Carro/Tustin Int3 ==
  In1 : Inport
  Gain : Gain  Gain=T_s/2
  Sum : Sum  Inputs=|++
  Sum1 : Sum  Inputs=|++
  Unit Delay : UnitDelay  SampleTime=T_s  HasFrameUpgradeWarning=on
  Unit Delay1 : UnitDelay  SampleTime=T_s  HasFrameUpgradeWarning=on
  Out1 : Outport
  wires:
  Sum1/1 -> Unit Delay/1, Out1/1
  Unit Delay/1 -> Sum1/2
  Unit Delay1/1 -> Sum/2
  In1/1 -> Sum/1, Unit Delay1/1
  Sum/1 -> Gain/1
  Gain/1 -> Sum1/1

== system modelo_f_nico_local/Nivel 2/Observador Carro/Tustin Int4 ==
  In1 : Inport
  Gain : Gain  Gain=T_s/2
  Sum : Sum  Inputs=|++
  Sum1 : Sum  Inputs=|++
  Unit Delay : UnitDelay  InitialCondition=theta_tm0  SampleTime=T_s  HasFrameUpgradeWarning=on
  Unit Delay1 : UnitDelay  SampleTime=T_s  HasFrameUpgradeWarning=on
  Out1 : Outport
  wires:
  Sum1/1 -> Unit Delay/1, Out1/1
  Unit Delay/1 -> Sum1/2
  Unit Delay1/1 -> Sum/2
  In1/1 -> Sum/1, Unit Delay1/1
  Sum/1 -> Gain/1
  Gain/1 -> Sum1/1

== system modelo_f_nico_local/Nivel 2/Observador Izaje/Tustin Int ==
  In1 : Inport
  Gain : Gain  Gain=T_s/2
  Sum : Sum  Inputs=|++
  Sum1 : Sum  Inputs=|++
  Unit Delay : UnitDelay  SampleTime=T_s  HasFrameUpgradeWarning=on
  Unit Delay1 : UnitDelay  SampleTime=T_s  HasFrameUpgradeWarning=on
  Out1 : Outport
  wires:
  Sum1/1 -> Unit Delay/1, Out1/1
  Unit Delay/1 -> Sum1/2
  Unit Delay1/1 -> Sum/2
  In1/1 -> Sum/1, Unit Delay1/1
  Sum/1 -> Gain/1
  Gain/1 -> Sum1/1

== system modelo_f_nico_local/Nivel 2/Observador Izaje/Tustin Int1 ==
  In1 : Inport
  Gain : Gain  Gain=T_s/2
  Sum : Sum  Inputs=|++
  Sum1 : Sum  Inputs=|++
  Unit Delay : UnitDelay  InitialCondition=theta_hm0  SampleTime=T_s  HasFrameUpgradeWarning=on
  Unit Delay1 : UnitDelay  SampleTime=T_s  HasFrameUpgradeWarning=on
  Out1 : Outport
  wires:
  Sum1/1 -> Unit Delay/1, Out1/1
  Unit Delay/1 -> Sum1/2
  Unit Delay1/1 -> Sum/2
  In1/1 -> Sum/1, Unit Delay1/1
  Sum/1 -> Gain/1
  Gain/1 -> Sum1/1

== system modelo_f_nico_local/Nivel 2/PID carro/Tustin Int1 ==
  In1 : Inport
  Gain : Gain  Gain=T_s/2
  Sum : Sum  Inputs=|++
  Sum1 : Sum  Inputs=|++
  Unit Delay : UnitDelay  SampleTime=T_s  HasFrameUpgradeWarning=on
  Unit Delay1 : UnitDelay  SampleTime=T_s  HasFrameUpgradeWarning=on
  Out1 : Outport
  wires:
  Sum1/1 -> Unit Delay/1, Out1/1
  Unit Delay/1 -> Sum1/2
  Unit Delay1/1 -> Sum/2
  In1/1 -> Sum/1, Unit Delay1/1
  Sum/1 -> Gain/1
  Gain/1 -> Sum1/1

== system modelo_f_nico_local/Nivel 2/PID carro/Tustin Int2 ==
  In1 : Inport
  Gain : Gain  Gain=T_s/2
  Sum : Sum  Inputs=|++
  Sum1 : Sum  Inputs=|++
  Unit Delay : UnitDelay  SampleTime=T_s  HasFrameUpgradeWarning=on
  Unit Delay1 : UnitDelay  SampleTime=T_s  HasFrameUpgradeWarning=on
  Out1 : Outport
  wires:
  Sum1/1 -> Unit Delay/1, Out1/1
  Unit Delay/1 -> Sum1/2
  Unit Delay1/1 -> Sum/2
  In1/1 -> Sum/1, Unit Delay1/1
  Sum/1 -> Gain/1
  Gain/1 -> Sum1/1

== system modelo_f_nico_local/Nivel 2/PID izaje/Tustin Int1 ==
  In1 : Inport
  Gain : Gain  Gain=T_s/2
  Sum : Sum  Inputs=|++
  Sum1 : Sum  Inputs=|++
  Unit Delay : UnitDelay  SampleTime=T_s  HasFrameUpgradeWarning=on
  Unit Delay1 : UnitDelay  SampleTime=T_s  HasFrameUpgradeWarning=on
  Out1 : Outport
  wires:
  Sum1/1 -> Unit Delay/1, Out1/1
  Unit Delay/1 -> Sum1/2
  Unit Delay1/1 -> Sum/2
  In1/1 -> Sum/1, Unit Delay1/1
  Sum/1 -> Gain/1
  Gain/1 -> Sum1/1

== system modelo_f_nico_local/Nivel 2/PID izaje/Tustin Int2 ==
  In1 : Inport
  Gain : Gain  Gain=T_s/2
  Sum : Sum  Inputs=|++
  Sum1 : Sum  Inputs=|++
  Unit Delay : UnitDelay  SampleTime=T_s  HasFrameUpgradeWarning=on
  Unit Delay1 : UnitDelay  SampleTime=T_s  HasFrameUpgradeWarning=on
  Out1 : Outport
  wires:
  Sum1/1 -> Unit Delay/1, Out1/1
  Unit Delay/1 -> Sum1/2
  Unit Delay1/1 -> Sum/2
  In1/1 -> Sum/1, Unit Delay1/1
  Sum/1 -> Gain/1
  Gain/1 -> Sum1/1

== system modelo_f_nico_local/Nivel 2/Subsistema físico/Accionamiento Carro ==
  T_tm : Inport
  F_tw : Inport  Port=2
  BRK_t : Inport  Port=3
  Gain : Gain  Gain=1/(J_tm_tb+J_td/i_t^2)
  Gain1 : Gain  Gain=r_td/i_t
  Gain2 : Gain  Gain=(b_tm+b_td/i_t^2)
  Integrator : Integrator  InitialCondition=w_tm0
  Integrator1 : Integrator  InitialCondition=theta_tm0
  Scope : Scope
  Subsystem : Subsystem
  Sum : Sum  Inputs=+-+-
  theta_tm : Outport
  w_tm : Outport  Port=2
  wires:
  Integrator1/1 -> theta_tm/1
  Integrator/1 -> w_tm/1, Gain2/1, Subsystem/2(w_tm), Integrator1/1  "w_tm"
  Gain/1 -> Integrator/1
  Sum/1 -> Gain/1
  T_tm/1 -> Sum/1
  F_tw/1 -> Gain1/1
  Gain1/1 -> Sum/2
  Subsystem/1(T_tb) -> Scope/1, Sum/3
  Gain2/1 -> Sum/4
  BRK_t/1 -> Subsystem/1(BRK_t)

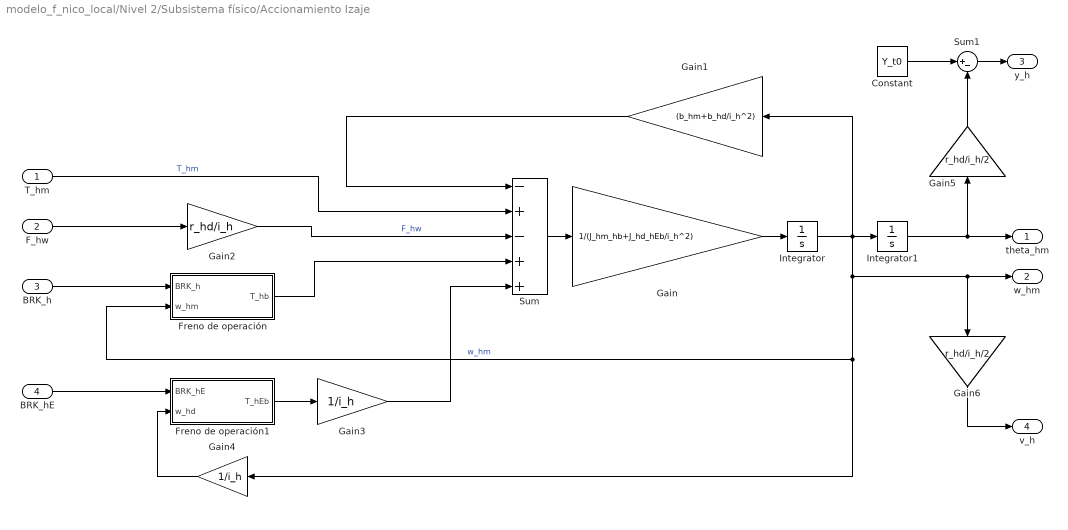
== system modelo_f_nico_local/Nivel 2/Subsistema físico/Accionamiento Izaje ==
  T_hm : Inport
  F_hw : Inport  Port=2
  BRK_h : Inport  Port=3
  BRK_hE : Inport  Port=4
  Constant : Constant  Value=Y_t0
  Freno de operación : Subsystem
  Freno de operación1 : Subsystem
  Gain : Gain  Gain=1/(J_hm_hb+J_hd_hEb/i_h^2)
  Gain1 : Gain  Gain=(b_hm+b_hd/i_h^2)
  Gain2 : Gain  Gain=r_hd/i_h
  Gain3 : Gain  Gain=1/i_h
  Gain4 : Gain  Gain=1/i_h
  Gain5 : Gain  Gain=r_hd/i_h/2
  Gain6 : Gain  Gain=r_hd/i_h/2
  Integrator : Integrator  InitialCondition=w_hm0
  Integrator1 : Integrator  InitialCondition=theta_hm0
  Sum : Sum  Inputs=-+-++
  Sum1 : Sum  Inputs=|+-
  theta_hm : Outport
  w_hm : Outport  Port=2
  y_h : Outport  Port=3
  v_h : Outport  Port=4
  wires:
  Integrator1/1 -> Gain5/1, theta_hm/1
  Integrator/1 -> Integrator1/1, Gain6/1, w_hm/1, Gain4/1, Freno de operación/2(w_hm), Gain1/1  "w_hm"
  Gain/1 -> Integrator/1
  Sum/1 -> Gain/1
  Gain1/1 -> Sum/1
  F_hw/1 -> Gain2/1
  Gain2/1 -> Sum/3  "F_hw"
  T_hm/1 -> Sum/2  "T_hm"
  Freno de operación/1(T_hb) -> Sum/4
  BRK_h/1 -> Freno de operación/1(BRK_h)
  Freno de operación1/1(T_hEb) -> Gain3/1
  Gain3/1 -> Sum/5
  BRK_hE/1 -> Freno de operación1/1(BRK_hE)
  Gain4/1 -> Freno de operación1/2(w_hd)
  Sum1/1 -> y_h/1
  Gain5/1 -> Sum1/2
  Constant/1 -> Sum1/1
  Gain6/1 -> v_h/1

== system modelo_f_nico_local/Nivel 2/Subsistema físico/Cable carro ==
  theta_tm : Inport
  w_tm : Inport  Port=2
  x_t : Inport  Port=3
  v_t : Inport  Port=4
  Gain : Gain  Gain=b_tw
  Gain1 : Gain  Gain=K_tw
  Gain2 : Gain  Gain=r_td/i_t
  Gain3 : Gain  Gain=r_td/i_t
  Sum : Sum  Inputs=|+-
  Sum1 : Sum  Inputs=|+-
  Sum2 : Sum  Inputs=|++
  F_tw : Outport
  wires:
  Sum/1 -> Gain1/1
  theta_tm/1 -> Gain3/1
  x_t/1 -> Sum/2
  Sum1/1 -> Gain/1
  w_tm/1 -> Gain2/1
  v_t/1 -> Sum1/2
  Gain/1 -> Sum2/2
  Gain1/1 -> Sum2/1
  Sum2/1 -> F_tw/1
  Gain2/1 -> Sum1/1  "v_td"
  Gain3/1 -> Sum/1  "x_td"

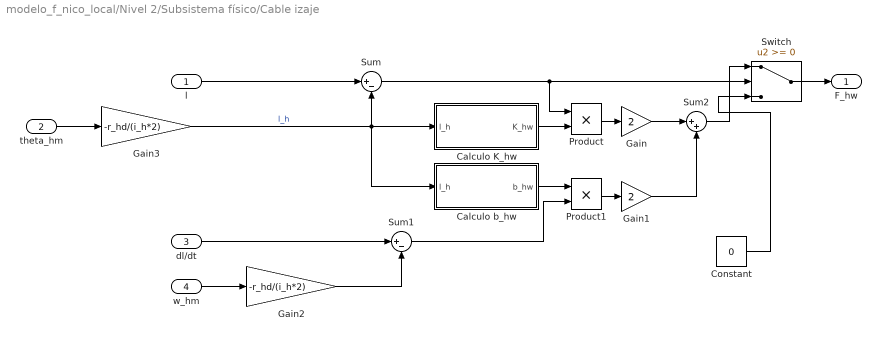
== system modelo_f_nico_local/Nivel 2/Subsistema físico/Cable izaje ==
  l : Inport
  theta_hm : Inport  Port=2
  dl/dt : Inport  Port=3
  w_hm : Inport  Port=4
  Calculo K_hw : Subsystem
  Calculo b_hw : Subsystem
  Constant : Constant  Value=0
  Gain : Gain  Gain=2
  Gain1 : Gain  Gain=2
  Gain2 : Gain  Gain=-r_hd/(i_h*2)
  Gain3 : Gain  Gain=-r_hd/(i_h*2)
  Product : Product
  Product1 : Product
  Sum : Sum  Inputs=|+-
  Sum1 : Sum  Inputs=|+-
  Sum2 : Sum  Inputs=|++
  Switch : Switch  SaturateOnIntegerOverflow=off  InputSameDT=off
  F_hw : Outport
  wires:
  l/1 -> Sum/1
  theta_hm/1 -> Gain3/1
  Sum/1 -> Product/1, Switch/2
  Calculo K_hw/1(K_hw) -> Product/2
  Product/1 -> Gain/1
  w_hm/1 -> Gain2/1
  Product1/1 -> Gain1/1
  Calculo b_hw/1(b_hw) -> Product1/1
  Gain1/1 -> Sum2/2
  Gain/1 -> Sum2/1
  Sum2/1 -> Switch/1
  Switch/1 -> F_hw/1
  dl/dt/1 -> Sum1/1
  Constant/1 -> Switch/3
  Gain2/1 -> Sum1/2
  Gain3/1 -> Calculo b_hw/1(l_h), Calculo K_hw/1(l_h), Sum/2  "l_h"
  Sum1/1 -> Product1/2

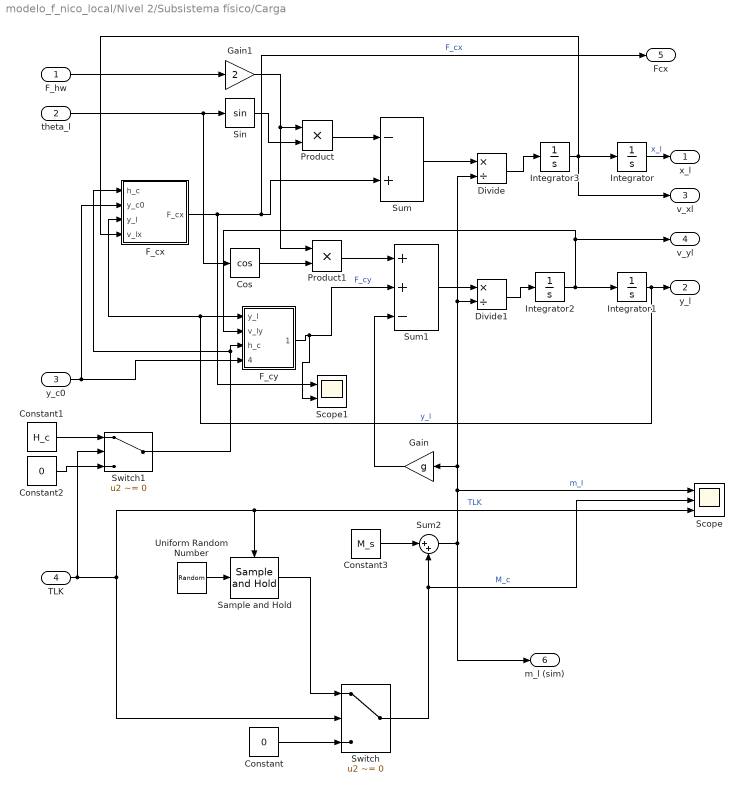
== system modelo_f_nico_local/Nivel 2/Subsistema físico/Carga ==
  F_hw : Inport
  theta_l : Inport  Port=2
  y_c0 : Inport  Port=3
  TLK : Inport  Port=4
  Constant : Constant  Value=0
  Constant1 : Constant  Value=H_c
  Constant2 : Constant  Value=0
  Constant3 : Constant  Value=M_s
  Cos : Trigonometry  Operator=cos
  Divide : Product  Inputs=*/
  Divide1 : Product  Inputs=*/
  F_cx : Subsystem
  F_cy : Subsystem
  Gain : Gain  Gain=g
  Gain1 : Gain  Gain=2
  Integrator : Integrator  InitialCondition=x_l0
  Integrator1 : Integrator  InitialCondition=y_l0
  Integrator2 : Integrator  InitialCondition=v_ly0
  Integrator3 : Integrator  InitialCondition=v_lx0
  Product : Product
  Product1 : Product
  Sample and Hold : dspsigops/Sample and Hold  trig=Rising edge  initCond=0  latchinput=off
  Scope : Scope  NumInputPorts=3
  Scope1 : Scope  NumInputPorts=2
  Sin : Trigonometry
  Sum : Sum  Inputs=-+
  Sum1 : Sum  Inputs=++-
  Sum2 : Sum  Inputs=|++
  Switch : Switch  Criteria=u2 ~= 0  SaturateOnIntegerOverflow=off  InputSameDT=off
  Switch1 : Switch  Criteria=u2 ~= 0  SaturateOnIntegerOverflow=off  InputSameDT=off
  Uniform Random Number : UniformRandomNumber  Minimum=M_cmin  Maximum=M_cmax  SampleTime=1
  x_l : Outport
  y_l : Outport  Port=2
  v_xl : Outport  Port=3
  v_yl : Outport  Port=4
  Fcx : Outport  Port=5
  m_l (sim) : Outport  Port=6
  wires:
  Sum/1 -> Divide/1
  Divide/1 -> Integrator3/1
  theta_l/1 -> Cos/1, Sin/1
  F_hw/1 -> Gain1/1
  Gain1/1 -> Product/1, Product1/1
  Sin/1 -> Product/2
  Product/1 -> Sum/1
  Switch1/1 -> F_cx/1(h_c), F_cy/3(h_c)
  Product1/1 -> Sum1/1
  Cos/1 -> Product1/2
  F_cy/1(F_cy) -> Scope1/2, Sum1/2  "F_cy"
  Divide1/1 -> Integrator2/1
  Sum1/1 -> Divide1/1
  Integrator/1 -> x_l/1  "x_l"
  Integrator3/1 -> v_xl/1, F_cx/4(v_lx), Integrator/1
  Integrator2/1 -> v_yl/1, F_cy/2(v_ly), Integrator1/1
  Integrator1/1 -> F_cx/3(y_l), F_cy/1(y_l), y_l/1  "y_l"
  y_c0/1 -> F_cx/2(y_c0), F_cy/4(y_c0)
  F_cx/1(F_cx) -> Scope1/1, Fcx/1, Sum/2  "F_cx"
  TLK/1 -> Switch1/2, Scope/3, Sample and Hold/Trigger, Switch/2  "TLK"
  Switch/1 -> Scope/2, Sum2/2  "M_c"
  Constant3/1 -> Sum2/1
  Sum2/1 -> Gain/1, Divide1/2, Divide/2, Scope/1, m_l (sim)/1  "m_l"
  Uniform Random Number/1 -> Sample and Hold/1
  Sample and Hold/1 -> Switch/1
  Constant/1 -> Switch/3
  Constant1/1 -> Switch1/1
  Constant2/1 -> Switch1/3
  Gain/1 -> Sum1/3

== system modelo_f_nico_local/Nivel 2/Subsistema físico/Carro ==
  F_tw : Inport
  theta_l : Inport  Port=2
  F_hw : Inport  Port=3
  Gain : Gain  Gain=2
  Gain1 : Gain  Gain=b_t
  Gain2 : Gain  Gain=1/M_t
  Integrator : Integrator  InitialCondition=v_t0
  Integrator1 : Integrator  InitialCondition=x_t0
  Product : Product
  Sin : Trigonometry
  Sum : Sum  Inputs=-++
  x_t : Outport
  v_t : Outport  Port=2
  wires:
  F_tw/1 -> Sum/3
  F_hw/1 -> Gain/1
  Gain/1 -> Product/1
  theta_l/1 -> Sin/1
  Sin/1 -> Product/2
  Product/1 -> Sum/2
  Integrator/1 -> v_t/1, Integrator1/1, Gain1/1  "v_t"
  Sum/1 -> Gain2/1
  Gain2/1 -> Integrator/1  "dv_t/dt"
  Integrator1/1 -> x_t/1
  Gain1/1 -> Sum/1

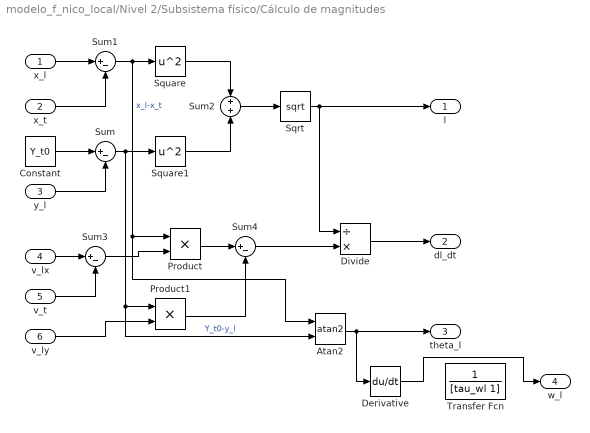
== system modelo_f_nico_local/Nivel 2/Subsistema físico/Cálculo de magnitudes ==
  x_l : Inport
  x_t : Inport  Port=2
  y_l : Inport  Port=3
  v_lx : Inport  Port=4
  v_t : Inport  Port=5
  v_ly : Inport  Port=6
  Atan2 : Trigonometry  Operator=atan2
  Constant : Constant  Value=Y_t0
  Derivative : Derivative
  Divide : Product  Inputs=/*
  Product : Product
  Product1 : Product
  Sqrt : Sqrt
  Square : Math  Operator=square
  Square1 : Math  Operator=square
  Sum{,1,3..4} (4 alike) : Sum  Inputs=|+-
  Sum2 : Sum  Inputs=+|+
  Transfer Fcn : TransferFcn  Denominator=[tau_wl 1]
  l : Outport
  dl_dt : Outport  Port=2
  theta_l : Outport  Port=3
  w_l : Outport  Port=4
  wires:
  Constant/1 -> Sum/1
  y_l/1 -> Sum/2
  x_l/1 -> Sum1/1
  x_t/1 -> Sum1/2
  Sum1/1 -> Atan2/1, Product/1, Square/1  "x_l-x_t"
  Sum/1 -> Atan2/2, Product1/1, Square1/1  "Y_t0-y_l"
  Square/1 -> Sum2/1
  Square1/1 -> Sum2/2
  Sum2/1 -> Sqrt/1
  Sqrt/1 -> Divide/1, l/1
  v_lx/1 -> Sum3/1
  v_t/1 -> Sum3/2
  Sum3/1 -> Product/2
  Product/1 -> Sum4/1
  v_ly/1 -> Product1/2
  Product1/1 -> Sum4/2
  Sum4/1 -> Divide/2
  Divide/1 -> dl_dt/1
  Atan2/1 -> Derivative/1, theta_l/1
  Derivative/1 -> w_l/1

== system modelo_f_nico_local/Nivel 2/Subsistema físico/Field Weaking Izaje ==
  w_hm : Inport
  Abs : Abs  SaturateOnIntegerOverflow=off
  Constant : Constant  Value=w_hm_rated
  Divide : Product  Inputs=*/
  Gain : Gain  Gain=T_hmMax
  Max : MinMax  Function=max  Inputs=2
  Square : Math  Operator=square
  T_hm_max : Outport
  wires:
  w_hm/1 -> Abs/1
  Constant/1 -> Divide/1, Max/2
  Divide/1 -> Square/1
  Square/1 -> Gain/1
  Gain/1 -> T_hm_max/1
  Abs/1 -> Max/1
  Max/1 -> Divide/2

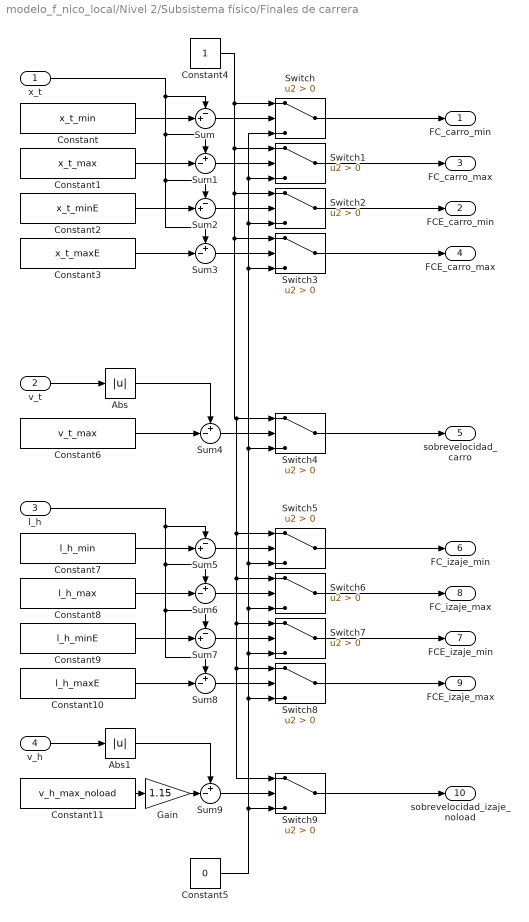
== system modelo_f_nico_local/Nivel 2/Subsistema físico/Finales de carrera ==
  x_t : Inport
  v_t : Inport  Port=2
  l_h : Inport  Port=3
  v_h : Inport  Port=4
  Abs : Abs  SaturateOnIntegerOverflow=off
  Abs1 : Abs  SaturateOnIntegerOverflow=off
  Constant : Constant  Value=x_t_min
  Constant1 : Constant  Value=x_t_max
  Constant10 : Constant  Value=l_h_maxE
  Constant11 : Constant  Value=v_h_max_noload
  Constant2 : Constant  Value=x_t_minE
  Constant3 : Constant  Value=x_t_maxE
  Constant4 : Constant
  Constant5 : Constant  Value=0
  Constant6 : Constant  Value=v_t_max
  Constant7 : Constant  Value=l_h_min
  Constant8 : Constant  Value=l_h_max
  Constant9 : Constant  Value=l_h_minE
  Gain : Gain  Gain=1.15
  Sum{,2,5,7} (4 alike) : Sum  Inputs=-+|
  Sum{1,3..4,6,8..9} (6 alike) : Sum  Inputs=+-|
  Switch{,1..9} (10 alike) : Switch  Criteria=u2 > Threshold  SaturateOnIntegerOverflow=off  InputSameDT=off
  FC_carro_min : Outport
  FCE_carro_min : Outport  Port=2
  FC_carro_max : Outport  Port=3
  FCE_carro_max : Outport  Port=4
  sobrevelocidad_carro : Outport  Port=5
  FC_izaje_min : Outport  Port=6
  FCE_izaje_min : Outport  Port=7
  FC_izaje_max : Outport  Port=8
  FCE_izaje_max : Outport  Port=9
  sobrevelocidad_izaje_noload : Outport  Port=10
  wires:
  Constant/1 -> Sum/2
  Constant1/1 -> Sum1/2
  Constant2/1 -> Sum2/2
  Constant3/1 -> Sum3/2
  x_t/1 -> Sum/1, Sum1/1, Sum2/1, Sum3/1
  Sum/1 -> Switch/2
  Constant4/1 -> Switch2/1, Switch9/1, Switch8/1, Switch7/1, Switch6/1, Switch5/1, Switch4/1, Switch3/1, Switch1/1, Switch/1
  Sum1/1 -> Switch1/2
  Sum2/1 -> Switch2/2
  Sum3/1 -> Switch3/2
  Switch/1 -> FC_carro_min/1
  Switch1/1 -> FC_carro_max/1
  Switch2/1 -> FCE_carro_min/1
  Switch3/1 -> FCE_carro_max/1
  v_t/1 -> Abs/1
  Constant6/1 -> Sum4/2
  Sum4/1 -> Switch4/2
  Abs/1 -> Sum4/1
  Switch4/1 -> sobrevelocidad_carro/1
  Switch7/1 -> FCE_izaje_min/1
  Switch6/1 -> FC_izaje_max/1
  l_h/1 -> Sum5/1, Sum6/1, Sum7/1, Sum8/1
  Sum7/1 -> Switch7/2
  Switch5/1 -> FC_izaje_min/1
  Constant7/1 -> Sum5/2
  Constant10/1 -> Sum8/2
  Constant9/1 -> Sum7/2
  Sum6/1 -> Switch6/2
  Constant8/1 -> Sum6/2
  Sum8/1 -> Switch8/2
  Constant5/1 -> Switch9/3, Switch8/3, Switch6/3, Switch5/3, Switch1/3, Switch/3, Switch2/3, Switch3/3, Switch4/3, Switch7/3
  Switch8/1 -> FCE_izaje_max/1
  Sum5/1 -> Switch5/2
  Constant11/1 -> Gain/1
  v_h/1 -> Abs1/1
  Abs1/1 -> Sum9/1
  Sum9/1 -> Switch9/2
  Switch9/1 -> sobrevelocidad_izaje_noload/1
  Gain/1 -> Sum9/2

== system modelo_f_nico_local/Nivel 2/Subsistema físico/Moduladores de torque ==
  T_tm* : Inport
  T_hm* : Inport  Port=2
  T_hmMax : Inport  Port=3
  +-T_tmMax : Saturate  UpperLimit=+T_tmMax  LowerLimit=-T_tmMax
  Gain : Gain  Gain=1/tau_tm
  Gain1 : Gain  Gain=1/tau_tm
  Gain2 : Gain  Gain=-1
  Integrator : Integrator
  Integrator1 : Integrator
  Saturation Dynamic : simulink/Discontinuities/Saturation Dynamic  OutMin=[]  OutMax=[]  OutDataTypeStr=Inherit: Same as second input  OutDataType=fixdt(1, 16)  OutScaling=2^-10  DoSatur=off
  Sum : Sum  Inputs=|+-
  Sum1 : Sum  Inputs=|+-
  T_tm : Outport
  T_hm : Outport  Port=2
  wires:
  +-T_tmMax/1 -> T_tm/1
  Gain/1 -> Integrator/1
  Integrator/1 -> Sum/2, +-T_tmMax/1
  T_tm*/1 -> Sum/1
  Sum/1 -> Gain/1
  Gain1/1 -> Integrator1/1
  Sum1/1 -> Gain1/1
  Integrator1/1 -> Sum1/2, Saturation Dynamic/2
  T_hm*/1 -> Sum1/1
  Saturation Dynamic/1 -> T_hm/1
  T_hmMax/1 -> Gain2/1, Saturation Dynamic/1
  Gain2/1 -> Saturation Dynamic/3

== system modelo_f_nico_local/Nivel 2/Subsistema físico/Accionamiento Carro/Subsystem ==
  BRK_t : Inport
  w_tm : Inport  Port=2
  Constant : Constant  Value=0
  Gain : Gain  Gain=b_tb
  Gain1 : Gain  Gain=-T_tbMax
  Switch : Switch  Criteria=u2 ~= 0  SaturateOnIntegerOverflow=off  InputSameDT=off
  Tanh : Trigonometry  Operator=tanh
  T_tb : Outport
  wires:
  BRK_t/1 -> Switch/2
  Constant/1 -> Switch/1
  Gain/1 -> Tanh/1
  w_tm/1 -> Gain/1
  Switch/1 -> T_tb/1
  Tanh/1 -> Gain1/1
  Gain1/1 -> Switch/3

== system modelo_f_nico_local/Nivel 2/Subsistema físico/Accionamiento Izaje/Freno de operación ==
  BRK_h : Inport
  w_hm : Inport  Port=2
  Constant : Constant  Value=0
  Gain : Gain  Gain=b_hb
  Gain1 : Gain  Gain=-T_hbMax
  Switch : Switch  Criteria=u2 ~= 0  SaturateOnIntegerOverflow=off  InputSameDT=off
  Tanh : Trigonometry  Operator=tanh
  T_hb : Outport
  wires:
  BRK_h/1 -> Switch/2
  Constant/1 -> Switch/1
  Gain/1 -> Tanh/1
  w_hm/1 -> Gain/1
  Switch/1 -> T_hb/1
  Tanh/1 -> Gain1/1
  Gain1/1 -> Switch/3

== system modelo_f_nico_local/Nivel 2/Subsistema físico/Accionamiento Izaje/Freno de operación1 ==
  BRK_hE : Inport
  w_hd : Inport  Port=2
  Constant : Constant  Value=0
  Gain : Gain  Gain=b_hd
  Gain1 : Gain  Gain=-T_hEbMax
  Switch : Switch  Criteria=u2 ~= 0  SaturateOnIntegerOverflow=off  InputSameDT=off
  Tanh : Trigonometry  Operator=tanh
  T_hEb : Outport
  wires:
  BRK_hE/1 -> Switch/2
  Constant/1 -> Switch/1
  Gain/1 -> Tanh/1
  w_hd/1 -> Gain/1
  Switch/1 -> T_hEb/1
  Tanh/1 -> Gain1/1
  Gain1/1 -> Switch/3

== system modelo_f_nico_local/Nivel 2/Subsistema físico/Cable izaje/Calculo K_hw ==
  l_h : Inport
  Constant : Constant  Value=110
  Constant1 : Constant  Value=k_wu
  Divide : Product  Inputs=*/
  Gain : Gain  Gain=2
  Sum : Sum  Inputs=|++
  K_hw : Outport
  wires:
  l_h/1 -> Gain/1
  Gain/1 -> Sum/1
  Constant/1 -> Sum/2
  Sum/1 -> Divide/2
  Constant1/1 -> Divide/1
  Divide/1 -> K_hw/1

== system modelo_f_nico_local/Nivel 2/Subsistema físico/Cable izaje/Calculo b_hw ==
  l_h : Inport
  Constant : Constant  Value=110
  Gain : Gain  Gain=2
  Gain1 : Gain  Gain=b_wu
  Sum : Sum  Inputs=|++
  b_hw : Outport
  wires:
  l_h/1 -> Gain/1
  Gain/1 -> Sum/1
  Constant/1 -> Sum/2
  Sum/1 -> Gain1/1
  Gain1/1 -> b_hw/1

== system modelo_f_nico_local/Nivel 2/Subsistema físico/Carga/F_cx ==
  h_c : Inport
  y_c0 : Inport  Port=2
  y_l : Inport  Port=3
  v_lx : Inport  Port=4
  Constant : Constant  Value=0
  Gain : Gain  Gain=-b_cx
  Sum : Sum  Inputs=|+-
  Sum1 : Sum  Inputs=|-+
  Switch : Switch  Criteria=u2 > Threshold  SaturateOnIntegerOverflow=off  InputSameDT=off
  F_cx : Outport
  wires:
  y_l/1 -> Sum/1
  h_c/1 -> Sum/2
  Sum/1 -> Sum1/1
  y_c0/1 -> Sum1/2
  Sum1/1 -> Switch/2
  Constant/1 -> Switch/3
  v_lx/1 -> Gain/1
  Gain/1 -> Switch/1
  Switch/1 -> F_cx/1
